simulink model "CDPR_INVERSKINEMATIKK_18_09_23"  (R2022b)
settings: Solver=FixedStepAuto  StartTime=0.0  StopTime=10.0  FixedStep=h  RelTol=1e-3
values from neighbouring files (symbols this model uses):
  a1 = A1 - origin    [CDPR_2R_test.m]    (also in CDPR_2T.m; TEST_INVERSKINEMATIKK.m = [0;1])
  a2 = A2 - origin    [CDPR_2R_test.m]    (also in CDPR_2T.m; TEST_INVERSKINEMATIKK.m = [1;1])
  a3 = A3 - origin    [CDPR_2R_test.m]    (also in CDPR_2T.m; TEST_INVERSKINEMATIKK.m = [0;0])
  a4 = A4 - origin    [CDPR_2R_test.m]    (also in CDPR_2T.m; TEST_INVERSKINEMATIKK.m = [1;0])
  b1 = B1 - body_origin    [CDPR_2R_test.m]    (also in CDPR_2T.m; TEST_INVERSKINEMATIKK.m = [0;L_end/2])
  b2 = B2 - body_origin    [CDPR_2R_test.m]    (also in CDPR_2T.m; TEST_INVERSKINEMATIKK.m = [0;-L_end/2])
  p = [0.5;0.5]    [TEST_INVERSKINEMATIKK.m]
  R = [cos(theta_body) -sin(theta_body);sin(theta_body) cos(theta_body)]    [TEST_INVERSKINEMATIKK.m]
settings Model: Creator=magag  LastModifiedBy=magngrot

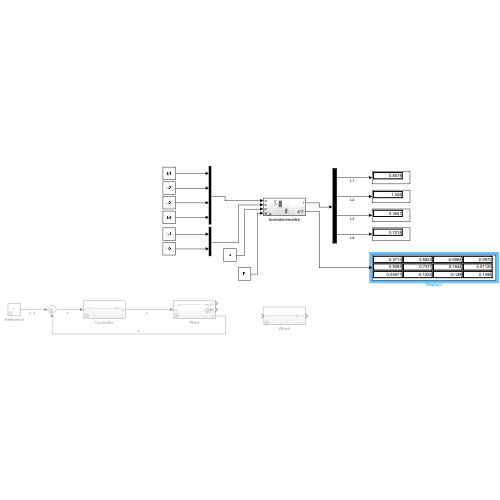
[thumbnail: Simulink's stored preview of the top-level diagram]
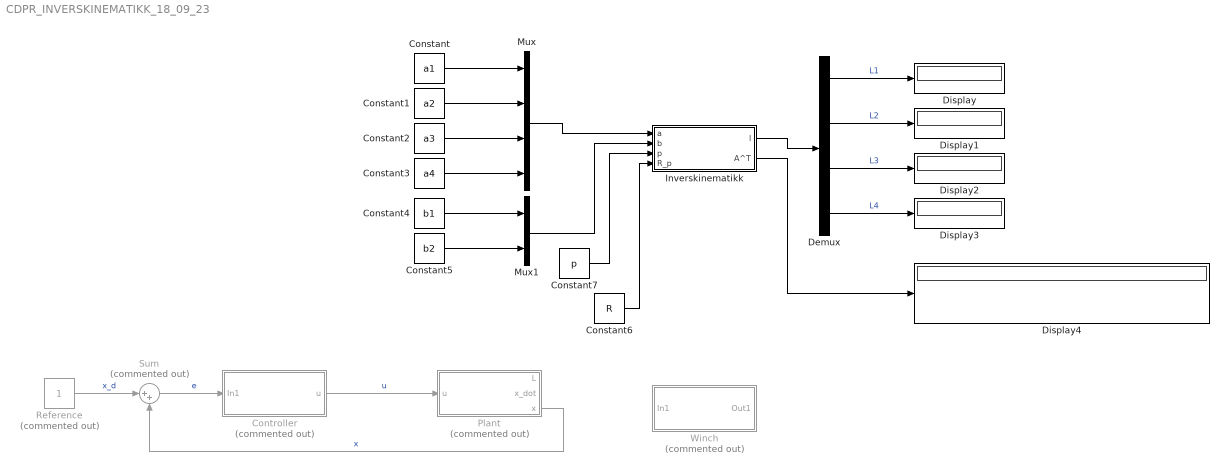
== system CDPR_INVERSKINEMATIKK_18_09_23 ==
  Constant : Constant  Value=a1
  Constant1 : Constant  Value=a2
  Constant2 : Constant  Value=a3
  Constant3 : Constant  Value=a4
  Constant4 : Constant  Value=b1
  Constant5 : Constant  Value=b2
  Constant6 : Constant  Value=R
  Constant7 : Constant  Value=p
  Controller : Subsystem  Commented=on
  Demux : Demux
  Display{,1..4} (5 alike) : Display
  Inverskinematikk : Subsystem
  Mux : Mux
  Mux1 : Mux  Inputs=2
  Plant : Subsystem  Commented=on
  Reference : Constant  Commented=on
  Sum : Sum  Commented=on  Inputs=|++
  Winch : Subsystem  Commented=on
  wires:
  Controller/1(u) -> Plant/1(u)  "u"
  Plant/3(x) -> Sum/2  "x"
  Reference/1 -> Sum/1  "x_d"
  Sum/1 -> Controller/1(In1)  "e"
  Constant/1 -> Mux/1
  Constant1/1 -> Mux/2
  Constant2/1 -> Mux/3
  Constant3/1 -> Mux/4
  Mux/1 -> Inverskinematikk/1(a)
  Constant4/1 -> Mux1/1
  Constant5/1 -> Mux1/2
  Mux1/1 -> Inverskinematikk/2(b)
  Inverskinematikk/1(l) -> Demux/1
  Demux/1 -> Display/1  "L1"
  Demux/2 -> Display1/1  "L2"
  Demux/3 -> Display2/1  "L3"
  Demux/4 -> Display3/1  "L4"
  Constant6/1 -> Inverskinematikk/4(R_p)
  Constant7/1 -> Inverskinematikk/3(p)
  Inverskinematikk/2(A^T) -> Display4/1

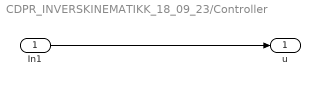
== system CDPR_INVERSKINEMATIKK_18_09_23/Controller ==
  In1 : Inport
  u : Outport
  wires:
  In1/1 -> u/1

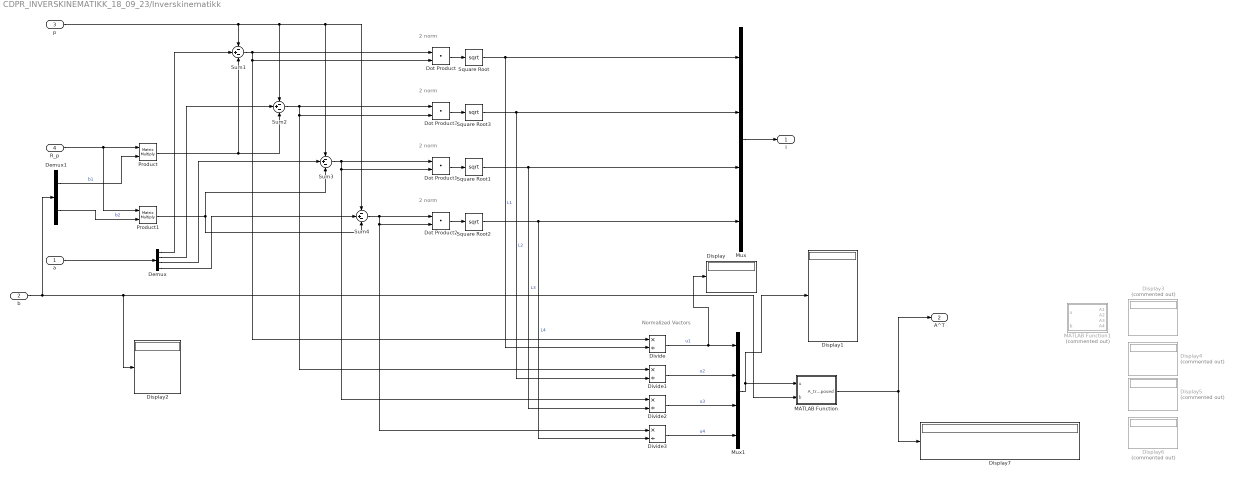
== system CDPR_INVERSKINEMATIKK_18_09_23/Inverskinematikk ==
  note: Normalized
      | Vectors
  note: 2 norm
  note: 2 norm
  note: 2 norm
  note: 2 norm
  a : Inport
  b : Inport  Port=2
  p : Inport  Port=3
  R_p : Inport  Port=4
  Demux : Demux
  Demux1 : Demux  Outputs=2
  Display{,1..2,7} (4 alike) : Display
  Display{3..6} (4 alike) : Display  Commented=on
  Divide{,1..3} (4 alike) : Product  Inputs=*/
  Dot Product{,1..3} (4 alike) : DotProduct  OutDataTypeStr=Inherit: Inherit via internal rule
  MATLAB Function : MATLAB Function  TreatAsAtomicUnit=on
  MATLAB Function1 : MATLAB Function  Commented=on  TreatAsAtomicUnit=on
  Mux : Mux
  Mux1 : Mux
  Product : Product  Multiplication=Matrix(*)
  Product1 : Product  Multiplication=Matrix(*)
  Square Root{,1..3} (4 alike) : Sqrt
  Sum{1..4} (4 alike) : Sum  Inputs=-+-
  l : Outport
  A^T : Outport  Port=2
  wires:
  R_p/1 -> Product/1, Product1/1
  Dot Product/1 -> Square Root/1
  a/1 -> Demux/1
  b/1 -> Demux1/1, Display2/1, MATLAB Function/2(b)
  Dot Product1/1 -> Square Root1/1
  Dot Product2/1 -> Square Root2/1
  Dot Product3/1 -> Square Root3/1
  Demux1/2 -> Product1/2  "b2"
  Demux1/1 -> Product/2  "b1"
  p/1 -> Sum3/1, Sum4/1, Sum2/1, Sum1/1
  Mux/1 -> l/1
  Demux/1 -> Sum1/2
  Demux/2 -> Sum2/2
  Demux/3 -> Sum3/2
  Demux/4 -> Sum4/2
  Product/1 -> Sum2/3, Sum1/3
  Product1/1 -> Sum3/3, Sum4/3
  Square Root/1 -> Divide/2, Mux/1  "L1"
  Square Root3/1 -> Mux/2, Divide1/2  "L2"
  Square Root1/1 -> Mux/3, Divide2/2  "L3"
  Square Root2/1 -> Mux/4, Divide3/2  "L4"
  Divide/1 -> Display/1, Mux1/1  "u1"
  Divide1/1 -> Mux1/2  "u2"
  Divide2/1 -> Mux1/3  "u3"
  Divide3/1 -> Mux1/4  "u4"
  Sum4/1 -> Dot Product2/1, Dot Product2/2, Divide3/1
  Sum1/1 -> Dot Product/1, Dot Product/2, Divide/1
  Sum2/1 -> Dot Product3/1, Dot Product3/2, Divide1/1
  Sum3/1 -> Dot Product1/1, Dot Product1/2, Divide2/1
  Mux1/1 -> Display1/1, MATLAB Function/1(u)
  MATLAB Function/1(A_transposed) -> A^T/1, Display7/1

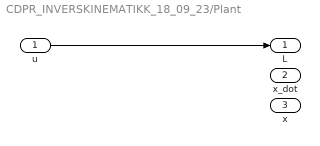
== system CDPR_INVERSKINEMATIKK_18_09_23/Plant ==
  u : Inport
  L : Outport
  x_dot : Outport  Port=2
  x : Outport  Port=3
  wires:
  u/1 -> L/1

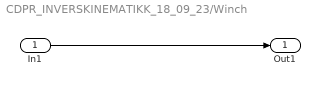
== system CDPR_INVERSKINEMATIKK_18_09_23/Winch ==
  In1 : Inport
  Out1 : Outport
  wires:
  In1/1 -> Out1/1

== matlab function CDPR_INVERSKINEMATIKK_18_09_23/Inverskinematikk/MATLAB Function1 ==
  data: u input; A1 output double size=3; b input; A2 output double; A3 output double; A4 output double
function [A1,A2,A3,A4] = fcn(u, b)
u1 = u(1:2);
u2 = u(3:4);
u3 = u(5:6);
u4 = u(7:8);
b1 = b(1:2);
b2 = b(3:4);

h1 = b1(1)*u1(2) - b1(2)*u1(1);
h2 = b1(1)*u2(2) - b1(2)*u2(1);
h3 = b2(1)*u3(2) - b2(2)*u3(1);
h4 = b2(1)*u4(2) - b2(2)*u4(1);

A1 = [u1;h1];
A2 = [u2;h2];
A3 = [u3;h3];
A4 = [u4;h4];

== matlab function CDPR_INVERSKINEMATIKK_18_09_23/Inverskinematikk/MATLAB Function ==
  data: u input; A_transposed output double; b input
function A_transposed = jacobi_A(u, b)
u1 = u(1:2);
u2 = u(3:4);
u3 = u(5:6);
u4 = u(7:8);
b1 = b(1:2);
b2 = b(3:4);

h1 = b1(1)*u1(2) - b1(2)*u1(1);
h2 = b1(1)*u2(2) - b1(2)*u2(1);
h3 = b2(1)*u3(2) - b2(2)*u3(1);
h4 = b2(1)*u4(2) - b2(2)*u4(1);

A1 = [u1;h1];
A2 = [u2;h2];
A3 = [u3;h3];
A4 = [u4;h4];

A_transposed = [A1 A2 A3 A4];
